simulink model "task1_1"  (R2024b)
settings: Solver=VariableStepAuto  StartTime=0.0  StopTime=4800  RelTol=1e-3
settings Model: Creator=User  LastModifiedBy=almansurkakimov
settings RTWCC: GPUComputeCapability=3.5

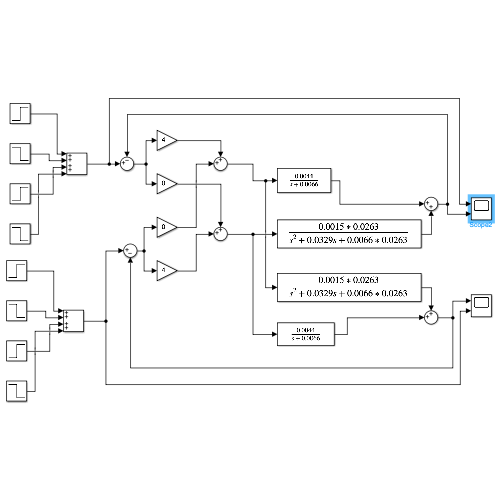
[thumbnail: Simulink's stored preview of the top-level diagram]
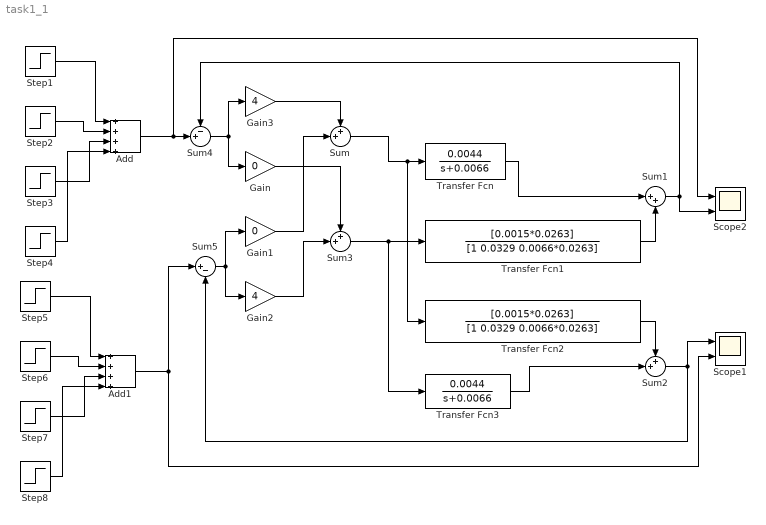
== system task1_1 ==
  Add : Sum  Inputs=++++
  Add1 : Sum  Inputs=++++
  Gain : Gain  Gain=0
  Gain1 : Gain  Gain=0
  Gain2 : Gain  Gain=4
  Gain3 : Gain  Gain=4
  Scope1 : Scope  NumInputPorts=2
  Scope2 : Scope  NumInputPorts=2
  Step1 : Step  Time=0  After=0.1  SampleTime=0
  Step2 : Step  Time=1200  After=-0.1  SampleTime=0
  Step3 : Step  Time=2400  After=0.1  SampleTime=0
  Step4 : Step  Time=3600  After=-0.1  SampleTime=0
  Step5 : Step  Time=600  After=0.1  SampleTime=0
  Step6 : Step  Time=1800  After=-0.1  SampleTime=0
  Step7 : Step  Time=3000  After=0.1  SampleTime=0
  Step8 : Step  Time=4200  After=-0.1  SampleTime=0
  Sum : Sum  Inputs=++|
  Sum1 : Sum  Inputs=|++
  Sum2 : Sum  Inputs=++|
  Sum3 : Sum  Inputs=++|
  Sum4 : Sum  Inputs=-+|
  Sum5 : Sum  Inputs=|+-
  Transfer Fcn : TransferFcn  Numerator=[0.0044]  Denominator=[1 0.0066]
  Transfer Fcn1 : TransferFcn  Numerator=[0.0015*0.0263]  Denominator=[1 0.0329 0.0066*0.0263]
  Transfer Fcn2 : TransferFcn  Numerator=[0.0015*0.0263]  Denominator=[1 0.0329 0.0066*0.0263]
  Transfer Fcn3 : TransferFcn  Numerator=[0.0044]  Denominator=[1 0.0066]
  wires:
  Add1/1 -> Sum5/1, Scope1/2
  Sum5/1 -> Gain2/1, Gain1/1
  Sum4/1 -> Gain/1, Gain3/1
  Sum/1 -> Transfer Fcn2/1, Transfer Fcn/1
  Sum3/1 -> Transfer Fcn3/1, Transfer Fcn1/1
  Gain3/1 -> Sum/1
  Gain1/1 -> Sum/2
  Gain2/1 -> Sum3/2
  Gain/1 -> Sum3/1
  Transfer Fcn/1 -> Sum1/1
  Transfer Fcn1/1 -> Sum1/2
  Sum1/1 -> Scope2/2, Sum4/1
  Sum2/1 -> Scope1/1, Sum5/2
  Transfer Fcn2/1 -> Sum2/1
  Transfer Fcn3/1 -> Sum2/2
  Step1/1 -> Add/1
  Step2/1 -> Add/2
  Step3/1 -> Add/3
  Step4/1 -> Add/4
  Add/1 -> Scope2/1, Sum4/2
  Step8/1 -> Add1/4
  Step7/1 -> Add1/3
  Step6/1 -> Add1/2
  Step5/1 -> Add1/1
